simulink model "MobileManipulatorSlave"  (R2016a)
settings: Solver=FixedStepAuto  SolverMode=SingleTasking  StartTime=0.0  StopTime=inf  FixedStep=.001  RelTol=1e-3
undefined symbols (not defined in the file): DiscIntNeverNeededParam, transl
libraries: simulink x20, LibrarySimulinkSAS x2, dspfactors x1, aerolibanimutils x1, dspnetwork x1
(part 2 of 2)

== matlab function MobileManipulatorSlave/REal /CONTROL system/Cinematica Inversa1/Jacobian1/jacob0 ==
  data: in1 input; out1 output
function out1 = jacob0(in1)
%#codegen

%    This function was generated by the Symbolic Math Toolbox version 6.1.
%    17-Aug-2017 11:26:19

q1 = in1(:,1);
q2 = in1(:,2);
q3 = in1(:,3);
q4 = in1(:,4);
q5 = in1(:,5);
q6 = in1(:,6);
q7 = in1(:,7);
t2 = cos(q1);
t3 = pi.*(1.0./2.0);
t4 = q6+t3;
t5 = cos(q4);
t6 = sin(q1);
t7 = sin(q3);
t8 = t6.*t7;
t9 = cos(q2);
t10 = cos(q3);
t15 = t2.*t9.*t10;
t11 = t8-t15;
t12 = sin(q2);
t13 = sin(q4);
t14 = sin(q5);
t16 = t5.*t11;
t17 = t2.*t12.*t13;
t18 = t16+t17;
t19 = cos(q5);
t20 = t6.*t10;
t21 = t2.*t7.*t9;
t22 = t20+t21;
t23 = cos(q7);
t24 = sin(q6);
t25 = cos(q6);
t26 = sin(q7);
t27 = cos(t4);
t28 = t11.*t13;
t34 = t2.*t5.*t12;
t29 = t28-t34;
t30 = sin(t4);
t31 = t18.*t19;
t32 = t14.*t22;
t33 = t31+t32;
t35 = t29.*t30;
t39 = t27.*t33;
t36 = t35-t39;
t37 = t14.*t18;
t41 = t19.*t22;
t38 = t37-t41;
t40 = t26.*t36;
t42 = t23.*t38;
t43 = t40+t42;
t44 = t27.*t29;
t45 = t30.*t33;
t46 = t44+t45;
t47 = t23.*t36;
t49 = t26.*t38;
t48 = t47-t49;
t50 = t2.*t7;
t51 = t6.*t9.*t10;
t52 = t50+t51;
t53 = t5.*t52;
t73 = t6.*t12.*t13;
t54 = t53-t73;
t55 = t2.*t10;
t75 = t6.*t7.*t9;
t56 = t55-t75;
t57 = t10.*t12.*t13.*t24.*8.0;
t58 = t7.*t12.*t14.*t25.*8.0;
t59 = t7.*t12.*t14.*t23.*1.7e1;
t60 = t5.*t7.*t12.*t14.*t23.*1.5e1;
t61 = t10.*t12.*t13.*t23.*t24.*8.0;
t62 = t7.*t12.*t14.*t23.*t25.*8.0;
t63 = t7.*t12.*t13.*t25.*t26.*1.5e1;
t64 = t10.*t12.*t14.*t24.*t26.*1.5e1;
t65 = t7.*t12.*t19.*t24.*t26.*1.7e1;
t66 = t9.*t13.*t14.*t24.*t26.*1.7e1;
t67 = t5.*t10.*t12.*t14.*t24.*t26.*1.7e1;
t68 = t5.*t7.*t12.*t19.*t24.*t26.*1.5e1;
t185 = t5.*t9.*t24.*8.0;
t186 = t9.*t13.*t19.*t25.*8.0;
t187 = t10.*t12.*t19.*t23.*1.5e1;
t188 = t9.*t13.*t19.*t23.*1.7e1;
t189 = t5.*t9.*t23.*t24.*8.0;
t190 = t5.*t10.*t12.*t19.*t25.*8.0;
t191 = t5.*t10.*t12.*t19.*t23.*1.7e1;
t192 = t9.*t13.*t19.*t23.*t25.*8.0;
t193 = t5.*t10.*t12.*t19.*t23.*t25.*8.0;
t69 = t57+t58+t59+t60+t61+t62+t63+t64+t65+t66+t67+t68-t185-t186-t187-t188-t189-t190-t191-t192-t193;
t70 = t13.*t52;
t71 = t5.*t6.*t12;
t72 = t70+t71;
t74 = t19.*t54;
t76 = t14.*t56;
t77 = t74+t76;
t78 = t7.*t12.*t19.*8.0;
t79 = t9.*t13.*t14.*8.0;
t80 = t5.*t10.*t12.*t14.*8.0;
t81 = t10.*t12.*t14.*t25.*1.5e1;
t82 = t7.*t12.*t19.*t25.*1.7e1;
t83 = t9.*t13.*t14.*t25.*1.7e1;
t84 = t7.*t12.*t19.*t23.*8.0;
t85 = t9.*t13.*t14.*t23.*8.0;
t86 = t5.*t10.*t12.*t14.*t25.*1.7e1;
t87 = t5.*t7.*t12.*t19.*t25.*1.5e1;
t88 = t5.*t10.*t12.*t14.*t23.*8.0;
t89 = t10.*t12.*t13.*t25.*t26.*8.0;
t90 = t9.*t13.*t19.*t24.*t26.*8.0;
t91 = t5.*t10.*t12.*t19.*t24.*t26.*8.0;
t210 = t5.*t9.*t25.*t26.*8.0;
t211 = t7.*t12.*t13.*t24.*1.5e1;
t212 = t7.*t12.*t14.*t24.*t26.*8.0;
t92 = t78+t79+t80+t81+t82+t83+t84+t85+t86+t87+t88+t89+t90+t91-t210-t211-t212;
t93 = t30.*t72;
t112 = t27.*t77;
t94 = t93-t112;
t95 = t14.*t54;
t110 = t19.*t56;
t96 = t95-t110;
t97 = t10.*t12.*t19.*t26.*1.5e1;
t98 = t9.*t13.*t19.*t26.*1.7e1;
t99 = t5.*t9.*t24.*t26.*8.0;
t100 = t5.*t10.*t12.*t19.*t26.*1.7e1;
t101 = t9.*t13.*t19.*t25.*t26.*8.0;
t102 = t7.*t12.*t13.*t23.*t25.*1.5e1;
t103 = t10.*t12.*t14.*t23.*t24.*1.5e1;
t104 = t7.*t12.*t19.*t23.*t24.*1.7e1;
t105 = t9.*t13.*t14.*t23.*t24.*1.7e1;
t106 = t5.*t10.*t12.*t19.*t25.*t26.*8.0;
t107 = t5.*t10.*t12.*t14.*t23.*t24.*1.7e1;
t108 = t5.*t7.*t12.*t19.*t23.*t24.*1.5e1;
t204 = t7.*t12.*t14.*t26.*1.7e1;
t205 = t5.*t7.*t12.*t14.*t26.*1.5e1;
t206 = t10.*t12.*t13.*t24.*t26.*8.0;
t207 = t7.*t12.*t14.*t25.*t26.*8.0;
t109 = t97+t98+t99+t100+t101+t102+t103+t104+t105+t106+t107+t108-t204-t205-t206-t207;
t111 = t23.*t96;
t113 = t26.*t94;
t114 = t111+t113;
t115 = t10.*t14.*t25.*8.0;
t116 = t10.*t14.*t23.*1.7e1;
t117 = t7.*t19.*t23.*1.5e1;
t118 = t5.*t7.*t19.*t25.*8.0;
t119 = t5.*t10.*t14.*t23.*1.5e1;
t120 = t5.*t7.*t19.*t23.*1.7e1;
t121 = t10.*t14.*t23.*t25.*8.0;
t122 = t10.*t13.*t25.*t26.*1.5e1;
t123 = t10.*t19.*t24.*t26.*1.7e1;
t124 = t5.*t7.*t19.*t23.*t25.*8.0;
t125 = t5.*t10.*t19.*t24.*t26.*1.5e1;
t215 = t7.*t13.*t24.*8.0;
t216 = t7.*t13.*t23.*t24.*8.0;
t217 = t7.*t14.*t24.*t26.*1.5e1;
t218 = t5.*t7.*t14.*t24.*t26.*1.7e1;
t126 = t115+t116+t117+t118+t119+t120+t121+t122+t123+t124+t125-t215-t216-t217-t218;
t127 = t27.*t72;
t128 = t30.*t77;
t129 = t127+t128;
t130 = t5.*t7.*t14.*8.0;
t131 = t10.*t13.*t24.*1.5e1;
t132 = t7.*t14.*t25.*1.5e1;
t133 = t5.*t7.*t14.*t25.*1.7e1;
t134 = t5.*t7.*t14.*t23.*8.0;
t135 = t7.*t13.*t25.*t26.*8.0;
t136 = t10.*t14.*t24.*t26.*8.0;
t137 = t5.*t7.*t19.*t24.*t26.*8.0;
t225 = t10.*t19.*8.0;
t226 = t10.*t19.*t25.*1.7e1;
t227 = t10.*t19.*t23.*8.0;
t228 = t5.*t10.*t19.*t25.*1.5e1;
t138 = t130+t131+t132+t133+t134+t135+t136+t137-t225-t226-t227-t228;
t139 = t23.*t94;
t156 = t26.*t96;
t140 = t139-t156;
t141 = t10.*t14.*t26.*1.7e1;
t142 = t7.*t19.*t26.*1.5e1;
t143 = t5.*t10.*t14.*t26.*1.5e1;
t144 = t5.*t7.*t19.*t26.*1.7e1;
t145 = t10.*t14.*t25.*t26.*8.0;
t146 = t7.*t14.*t23.*t24.*1.5e1;
t147 = t5.*t7.*t19.*t25.*t26.*8.0;
t148 = t5.*t7.*t14.*t23.*t24.*1.7e1;
t232 = t10.*t13.*t23.*t25.*1.5e1;
t233 = t10.*t19.*t23.*t24.*1.7e1;
t234 = t7.*t13.*t24.*t26.*8.0;
t235 = t5.*t10.*t19.*t23.*t24.*1.5e1;
t149 = t141+t142+t143+t144+t145+t146+t147+t148-t232-t233-t234-t235;
t150 = t5.*t24.*8.0;
t151 = t13.*t19.*t25.*8.0;
t152 = t13.*t19.*t23.*1.7e1;
t153 = t5.*t23.*t24.*8.0;
t154 = t13.*t19.*t23.*t25.*8.0;
t238 = t13.*t14.*t24.*t26.*1.7e1;
t155 = t150+t151+t152+t153+t154-t238;
t157 = t13.*t19.*t26.*1.7e1;
t158 = t5.*t24.*t26.*8.0;
t159 = t13.*t19.*t25.*t26.*8.0;
t160 = t13.*t14.*t23.*t24.*1.7e1;
t161 = t157+t158+t159+t160;
t162 = t13.*t14.*8.0;
t163 = t13.*t14.*t25.*1.7e1;
t164 = t13.*t14.*t23.*8.0;
t165 = t13.*t19.*t24.*t26.*8.0;
t236 = t5.*t25.*t26.*8.0;
t166 = t162+t163+t164+t165-t236;
t167 = t14.*t26.*1.7e1;
t168 = t14.*t25.*t26.*8.0;
t239 = t19.*t23.*t24.*1.7e1;
t169 = t167+t168-t239;
t170 = t14.*t25.*8.0;
t171 = t14.*t23.*1.7e1;
t172 = t14.*t23.*t25.*8.0;
t173 = t19.*t24.*t26.*1.7e1;
t174 = t170+t171+t172+t173;
t175 = t19.*8.0;
t176 = t19.*t25.*1.7e1;
t177 = t19.*t23.*8.0;
t240 = t14.*t24.*t26.*8.0;
t178 = t175+t176+t177-t240;
t179 = t23+1.0;
t180 = t23.*8.0;
t181 = t180+8.0;
t182 = t9.*t13;
t183 = t5.*t10.*t12;
t184 = t182+t183;
t194 = t14.*t184;
t195 = t7.*t12.*t19;
t196 = t194+t195;
t197 = t19.*t184;
t208 = t7.*t12.*t14;
t198 = t197-t208;
t199 = t27.*t198;
t200 = t5.*t9;
t209 = t10.*t12.*t13;
t201 = t200-t209;
t202 = t30.*t201;
t203 = t199+t202;
t213 = t23.*t196;
t237 = t26.*t203;
t214 = t213-t237;
t219 = t9.*t13.*t19;
t220 = t5.*t10.*t12.*t19;
t221 = -t208+t219+t220;
t222 = t25.*t221;
t223 = t24.*t201;
t224 = t222+t223;
t229 = t26.*t196;
t230 = t23.*t203;
t231 = t229+t230;
t241 = t13.*t23.*t25;
t242 = t5.*t19.*t23.*t24;
t276 = t5.*t14.*t26;
t243 = t241+t242-t276;
t244 = t19.*t26;
t245 = t14.*t23.*t24;
t246 = t244+t245;
t247 = t5.*t14.*t23;
t248 = t13.*t25.*t26;
t249 = t5.*t19.*t24.*t26;
t250 = t247+t248+t249;
t251 = t19.*t23;
t262 = t14.*t24.*t26;
t252 = t251-t262;
t253 = t13.*t14.*t26;
t254 = t5.*t23.*t25;
t274 = t13.*t19.*t23.*t24;
t255 = t253+t254-t274;
t256 = t13.*t14.*t23;
t257 = t13.*t19.*t24.*t26;
t263 = t5.*t25.*t26;
t258 = t256+t257-t263;
t259 = t5.*t24;
t260 = t13.*t19.*t25;
t261 = t259+t260;
t264 = t9.*t258;
t265 = t10.*t250;
t266 = t7.*t252;
t267 = t265+t266;
t268 = t12.*t267;
t269 = t264+t268;
t270 = t10.*t13.*t24;
t271 = t7.*t14.*t25;
t289 = t5.*t10.*t19.*t25;
t272 = t270+t271-t289;
t273 = t9.*t261;
t275 = t9.*t255;
t277 = t7.*t246;
t288 = t10.*t243;
t278 = t12.*(t277-t288);
t279 = t275+t278;
t280 = t7.*t243;
t281 = t10.*t246;
t282 = t280+t281;
t283 = t7.*t250;
t291 = t10.*t252;
t284 = t283-t291;
t285 = t10.*t14.*t25;
t286 = t5.*t7.*t19.*t25;
t290 = t7.*t13.*t24;
t287 = t285+t286-t290;
out1 = reshape([t43.*t69+t46.*t92+t48.*t109,-t69.*t114-t92.*t129-t109.*t140,-t69.*t214-t92.*t224+t109.*t231,-t43.*t269+t48.*t279-t46.*(t273-t12.*t272),t114.*t269-t140.*t279+t129.*(t273-t12.*t272),t214.*t269+t231.*t279+t224.*(t273-t12.*t272),t43.*t126-t46.*t138-t48.*t149,-t114.*t126+t129.*t138+t140.*t149,-t126.*t214+t138.*t224-t149.*t231,t43.*t284+t48.*t282+t46.*t287,-t114.*t284-t129.*t287-t140.*t282,-t214.*t284-t224.*t287+t231.*t282,-t43.*t155+t48.*t161+t46.*t166,t114.*t155-t129.*t166-t140.*t161,t155.*t214-t166.*t224+t161.*t231,-t43.*t258+t48.*t255-t46.*t261,t114.*t258+t129.*t261-t140.*t255,t214.*t258+t224.*t261+t231.*t255,t43.*t174-t48.*t169+t46.*t178,-t114.*t174-t129.*t178+t140.*t169,-t174.*t214-t169.*t231-t178.*t224,t48.*t246-t43.*t252+t14.*t25.*t46,t114.*t252-t140.*t246-t14.*t25.*t129,t214.*t252+t231.*t246-t14.*t25.*t224,t25.*t26.*t46.*-8.0+t24.*t26.*t48.*8.0-t24.*t43.*t179.*8.0,t25.*t26.*t129.*8.0-t24.*t26.*t140.*8.0+t24.*t114.*t179.*8.0,t25.*t26.*t224.*8.0+t24.*t26.*t231.*8.0+t24.*t179.*t214.*8.0,-t24.*t46+t25.*t26.*t43+t23.*t25.*t48,t24.*t129-t25.*t26.*t114-t23.*t25.*t140,t24.*t224-t25.*t26.*t214+t23.*t25.*t231,t46.*t181,-t129.*t181,-t181.*t224,-t23.*t43+t26.*t48,t23.*t114-t26.*t140,t23.*t214+t26.*t231,t23.*t38.*-8.0-t26.*t36.*8.0,t23.*t96.*8.0+t26.*t94.*8.0,t23.*t196.*8.0-t26.*t203.*8.0,-t44-t45,t129,t224],[6, 7]);

== matlab function MobileManipulatorSlave/REal /CONTROL system/Cinematica Inversa1/MATLAB Function2 ==
  data: J input; N output
function N = Null(J)
Jp=pinv(J);
I=eye(length(J));
N=(I-Jp*J)';

== matlab function MobileManipulatorSlave/REal /CONTROL system/Cinematica Inversa1/Metodo Cinematico Inverso/Inversa sin singularidad/Inversa Segura ==
  data: u input; y output
function y = fcn(u)

n=length(u);
invu=zeros(n,1);
for i=1:n
    if(abs(u(i))>0.005)
        invu(i)=1/u(i);
    else
        invu(i)=0;
    end
end

y=diag(invu);
